simulink model "two_tank_sandbox"  (R2016a)
settings: Solver=VariableStepAuto  StartTime=0.0  StopTime=15.0  RelTol=1e-3
libraries: tank_model x3
settings Model: Creator=Ibrahim  LastModifiedBy=Ibrahim

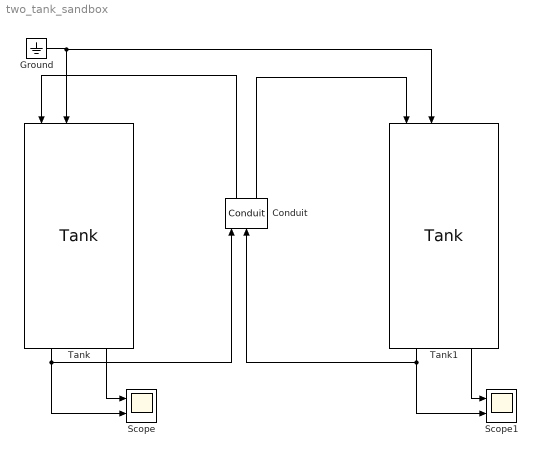
== system two_tank_sandbox ==
  Conduit : tank_model/Conduit  R=10  constI=on  I=-10
  Ground : Ground
  Scope : Scope  NumInputPorts=2
  Scope1 : Scope  NumInputPorts=2
  Tank : tank_model/Tank  C=10  V0=10  R=2  Vmax=100
  Tank1 : tank_model/Tank  C=5  V0=20  R=2  Vmax=100
  wires:
  Ground/1 -> Tank1/2, Tank/2
  Tank/1 -> Scope/2, Conduit/1
  Tank1/1 -> Scope1/2, Conduit/2
  Conduit/2 -> Tank1/1
  Conduit/1 -> Tank/1
  Tank/2 -> Scope/1
  Tank1/2 -> Scope1/1
